simulink model "Pendulo"  (R2018b)
settings: Solver=ode113  StartTime=0.0  StopTime=30  RelTol=1e-3
values from neighbouring files (symbols this model uses):
  A = [0 0 0 -0.0317 1 0 0 21.98 0 1 0 6.892 ... (16 elements, 4x4)]    [funcionalead.mat]    (also in pendulo.m = [0 1 0 0;0 0 1 0; 0 0 0 1; -.0317 21.98 6.892 0]; system1 funcionando.mat; system1.mat)
  B = [0 0 0 1]    [funcionalead.mat]    (also in pendulo.m = [0 0 0 1]'; system1 funcionando.mat; system1.mat)
  C = [-68.91 0 3.616 0]    [funcionalead.mat]    (also in pendulo.m; system1 funcionando.mat; system1.mat = [1 0 0 0])
  K = [119.9683 175.98 77.892 14]    [funcionalead.mat]    (also in system1 funcionando.mat; system1.mat)
undefined symbols (not defined in the file or in its folder): A3, B3, C3, K3, K3B, L3
libraries: cstblocks x1
settings Model: Creator=Abraham Pérez  LastModifiedBy=Abraham Pérez
settings SolverCC: InitialStep=.001

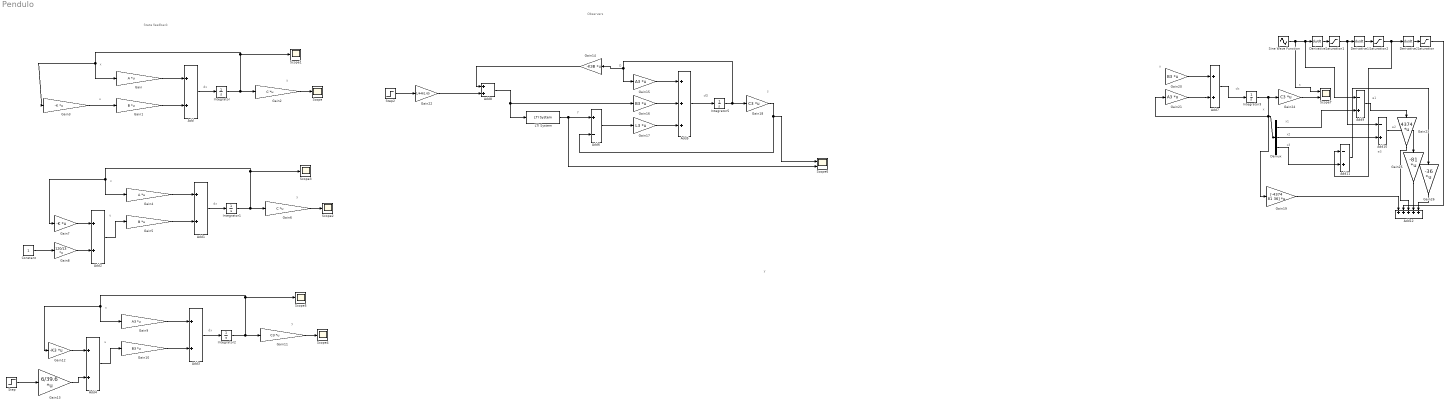
== system Pendulo ==
  note: e3
  note: e2
  note: e1
  note: x3
  note: x2
  note: x1
  note: x
  note: u
  note: State feedback
  note: y
  note: dx
  note: u
  note: x
  note: dx
  note: y
  note: x
  note: u
  note: dx
  note: x
  note: y
  note: u
  note: Observers
  note: dO
  note: y
  note: s
  note: y
  note: O
  note: s
  note: dx
  Add{,1..4,7..8} (7 alike) : Sum
  Add10 : Sum  Inputs=-+
  Add11 : Sum  Inputs=-+
  Add12 : Sum  Inputs=+++++
  Add5 : Sum  Inputs=+++
  Add6 : Sum  Inputs=+-
  Add9 : Sum  Inputs=-+
  Constant : Constant
  Demux : Demux  Outputs=3
  Derivative : Derivative
  Derivative1 : Derivative
  Derivative2 : Derivative
  Gain : Gain  Gain=A  Multiplication=Matrix(K*u)
  Gain1 : Gain  Gain=B  Multiplication=Matrix(K*u)
  Gain10 : Gain  Gain=B3  Multiplication=Matrix(K*u)
  Gain11 : Gain  Gain=C3  Multiplication=Matrix(K*u)
  Gain12 : Gain  Gain=-K3  Multiplication=Matrix(K*u)
  Gain13 : Gain  Gain=6/39.6  Multiplication=Matrix(K*u)
  Gain14 : Gain  Gain=-K3B  Multiplication=Matrix(K*u)
  Gain15 : Gain  Gain=A3  Multiplication=Matrix(K*u)
  Gain16 : Gain  Gain=B3  Multiplication=Matrix(K*u)
  Gain17 : Gain  Gain=L3  Multiplication=Matrix(K*u)
  Gain18 : Gain  Gain=C3  Multiplication=Matrix(K*u)
  Gain19 : Gain  Gain=[-4374 81 36]  Multiplication=Matrix(K*u)
  Gain2 : Gain  Gain=C  Multiplication=Matrix(K*u)
  Gain20 : Gain  Gain=B3  Multiplication=Matrix(K*u)
  Gain21 : Gain  Gain=A3  Multiplication=Matrix(K*u)
  Gain22 : Gain  Gain=1/4461.65
  Gain23 : Gain  Gain=4374  Multiplication=Matrix(K*u)
  Gain24 : Gain  Gain=C3  Multiplication=Matrix(K*u)
  Gain25 : Gain  Gain=-81  Multiplication=Matrix(K*u)
  Gain26 : Gain  Gain=-36  Multiplication=Matrix(K*u)
  Gain3 : Gain  Gain=-K  Multiplication=Matrix(K*u)
  Gain4 : Gain  Gain=A  Multiplication=Matrix(K*u)
  Gain5 : Gain  Gain=B  Multiplication=Matrix(K*u)
  Gain6 : Gain  Gain=C  Multiplication=Matrix(K*u)
  Gain7 : Gain  Gain=-K  Multiplication=Matrix(K*u)
  Gain8 : Gain  Gain=120/13  Multiplication=Matrix(K*u)
  Gain9 : Gain  Gain=A3  Multiplication=Matrix(K*u)
  Integrator : Integrator  InitialCondition=[-1 .5 .5 1]
  Integrator1 : Integrator  InitialCondition=[-1 .5 .5 1]
  Integrator2 : Integrator  InitialCondition=[-1 .5 .5 ]
  Integrator3 : Integrator  InitialCondition=[1 0 -1]
  Integrator5 : Integrator  InitialCondition=[1 0 -1]
  LTI System : cstblocks/LTI System  sys=G3  IC=[]
  Saturation : Saturate  UpperLimit=1  LowerLimit=-1
  Saturation1 : Saturate  UpperLimit=1  LowerLimit=-1
  Saturation2 : Saturate  UpperLimit=1  LowerLimit=-1
  Scope{,1..5} (6 alike) : Scope
  Scope6 : Scope  NumInputPorts=2
  Scope7 : Scope  NumInputPorts=2
  Sine Wave Function : Sin  TimeSource=Use external signal  SampleTime=0
  Step : Step  After=26  SampleTime=0
  Step2 : Step  After=26  SampleTime=0
  wires:
  Integrator/1 -> Gain2/1, Scope1/1, Gain/1, Gain3/1
  Gain/1 -> Add/1
  Gain1/1 -> Add/2
  Add/1 -> Integrator/1
  Gain2/1 -> Scope/1
  Gain3/1 -> Gain1/1
  Add1/1 -> Integrator1/1
  Integrator1/1 -> Gain6/1, Scope3/1, Gain4/1, Gain7/1
  Gain5/1 -> Add1/2
  Gain6/1 -> Scope2/1
  Gain4/1 -> Add1/1
  Gain7/1 -> Add2/1
  Add2/1 -> Gain5/1
  Gain8/1 -> Add2/2
  Constant/1 -> Gain8/1
  Step/1 -> Gain13/1
  Gain12/1 -> Add4/1
  Gain13/1 -> Add4/2
  Add4/1 -> Gain10/1
  Gain10/1 -> Add3/2
  Gain11/1 -> Scope4/1
  Gain9/1 -> Add3/1
  Add3/1 -> Integrator2/1
  Integrator2/1 -> Gain11/1, Scope5/1, Gain9/1, Gain12/1
  Gain17/1 -> Add5/3
  LTI System/1 -> Scope6/2, Add6/1
  Add6/1 -> Gain17/1
  Integrator5/1 -> Gain18/1, Gain15/1, Gain14/1
  Add5/1 -> Integrator5/1
  Gain15/1 -> Add5/1
  Gain16/1 -> Add5/2
  Gain14/1 -> Add8/1
  Gain22/1 -> Add8/2
  Step2/1 -> Gain22/1
  Add8/1 -> Gain16/1, LTI System/1
  Gain18/1 -> Scope6/1, Add6/2
  Gain20/1 -> Add7/1
  Add7/1 -> Integrator3/1
  Gain21/1 -> Add7/2
  Sine Wave Function/1 -> Derivative/1, Add9/1, Scope7/1
  Derivative1/1 -> Saturation2/1
  Gain24/1 -> Scope7/2
  Demux/1 -> Add9/2
  Demux/2 -> Add10/2
  Demux/3 -> Add11/2
  Integrator3/1 -> Gain19/1, Gain21/1, Demux/1, Gain24/1
  Gain19/1 -> Add12/1
  Add9/1 -> Gain23/1
  Gain23/1 -> Add12/3
  Add10/1 -> Gain25/1
  Gain25/1 -> Add12/4
  Add11/1 -> Gain26/1
  Gain26/1 -> Add12/5
  ? -> Gain20/1
  Derivative2/1 -> Saturation/1
  Saturation2/1 -> Add11/1, Derivative2/1
  Derivative/1 -> Saturation1/1
  Saturation1/1 -> Add10/1, Derivative1/1
  Saturation/1 -> Add12/2
